simulink model "pos_id_step_sl"  (Simulink 7.9)
settings: Solver=FixedStepDiscrete  StartTime=0.0  StopTime=tfinal  FixedStep=ts  RelTol=1e-3
values from neighbouring files (symbols this model uses):
  Kp_id = 0.12    [pos_id_step.m]
  r = 60    [pos_id_step.m]    (also in pos_pd_mbd.m; pos_pid2_mbd.m; pos_pid_mbd.m; pos_pid_set.m)
  r_cyc = 8    [pos_id_step.m]    (also in pos_pd_mbd.m = 4; pos_pid2_mbd.m = 4; pos_pid_mbd.m = 4; pos_pid_set.m = 4)
  ts = 1/50    (= 0.02)    [sim_init.m]    (also in sim_param.mat)
libraries: arduino_io_lib x5
settings Model: Creator=hirata  LastModifiedBy=hirata
settings DebuggingCC: FcnCallInpInsideContextMsg=Use local settings
settings GRTTargetCC: CombineOutputUpdateFcns=off  GRTInterface=on

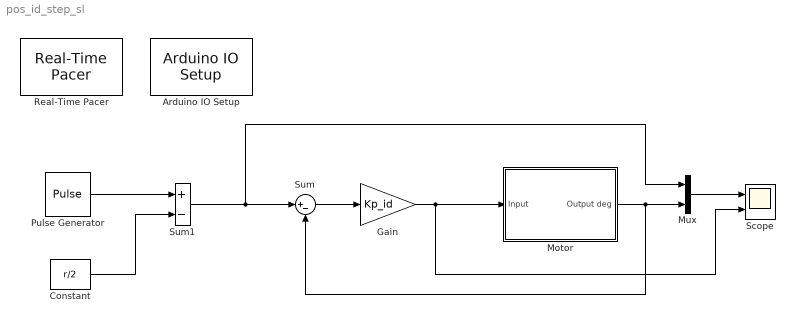
== system pos_id_step_sl ==
  Arduino IO Setup : arduino_io_lib/Arduino IO Setup  Priority=3  arduinoVar=Temporary arduino variable: Arduino1  workspaceVarName=a  comPort=COM3
  Constant : Constant  Value=r/2
  Gain : Gain  Gain=Kp_id
  Motor : Subsystem
  Mux : Mux  Inputs=2
  Pulse Generator : DiscretePulseGenerator  PulseType=Time based  Amplitude=r  Period=r_cyc  PulseWidth=50
  Real-Time Pacer : arduino_io_lib/Real-Time Pacer  simTimePerRealTime=1
  Scope : Scope  NumInputPorts=2
      settings: TimeRange=8  YMin=-80~-5  YMax=80~5  SaveName=yout
  Sum : Sum  Inputs=|+-
  Sum1 : Sum  Inputs=+-
  wires:
  Gain/1 -> Motor/1(Input), Scope/2
  Sum/1 -> Gain/1
  Sum1/1 -> Sum/1, Mux/1
  Motor/1(Output deg) -> Sum/2, Mux/2
  Pulse Generator/1 -> Sum1/1
  Constant/1 -> Sum1/2
  Mux/1 -> Scope/1

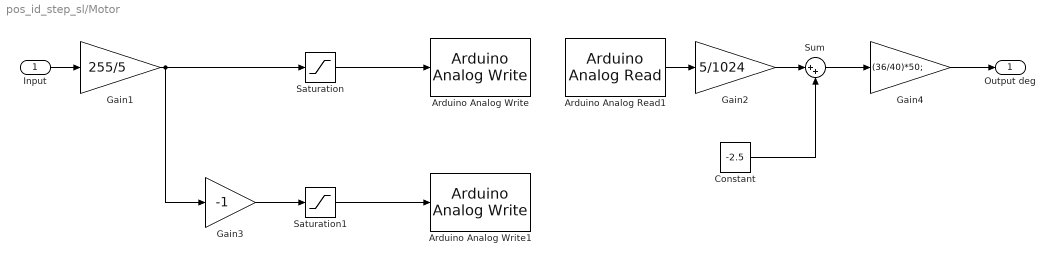
== system pos_id_step_sl/Motor ==
  Input : Inport
  Arduino Analog Read1 : arduino_io_lib/Arduino Analog Read  arduinoVar=Temporary arduino variable: Arduino1  arduinoPin=0  T=ts
  Arduino Analog Write : arduino_io_lib/Arduino Analog Write  arduinoVar=Temporary arduino variable: Arduino1  arduinoPin=3  T=ts
  Arduino Analog Write1 : arduino_io_lib/Arduino Analog Write  arduinoVar=Temporary arduino variable: Arduino1  arduinoPin=5  T=ts
  Constant : Constant  Value=-2.5
  Gain1 : Gain  Gain=255/5
  Gain2 : Gain  Gain=5/1024
  Gain3 : Gain  Gain=-1
  Gain4 : Gain  Gain=(36/40)*50;
  Saturation : Saturate  UpperLimit=255  LowerLimit=0
  Saturation1 : Saturate  UpperLimit=255  LowerLimit=0
  Sum : Sum  Inputs=|++
  Output deg : Outport
  wires:
  Input/1 -> Gain1/1
  Arduino Analog Read1/1 -> Gain2/1
  Saturation/1 -> Arduino Analog Write/1
  Gain1/1 -> Gain3/1, Saturation/1
  Saturation1/1 -> Arduino Analog Write1/1
  Gain4/1 -> Output deg/1
  Gain2/1 -> Sum/1
  Sum/1 -> Gain4/1
  Constant/1 -> Sum/2
  Gain3/1 -> Saturation1/1
